simulink model "IeI"  (R2022a)
settings: Solver=FixedStepAuto  StartTime=0.0  StopTime=100000  FixedStep=0.01  RelTol=1e-3
libraries: cstblocks x3
settings Model: Creator=loryb  LastModifiedBy=loryb

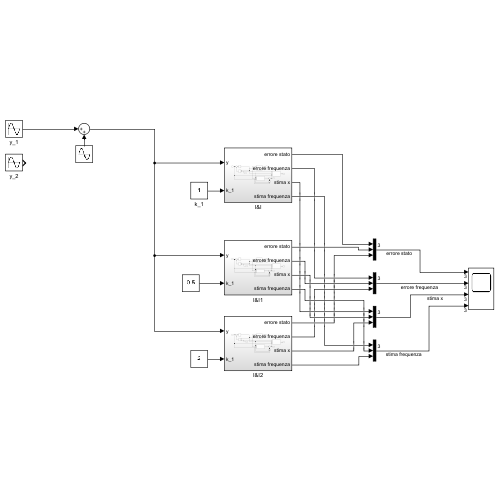
[thumbnail: Simulink's stored preview of the top-level diagram]
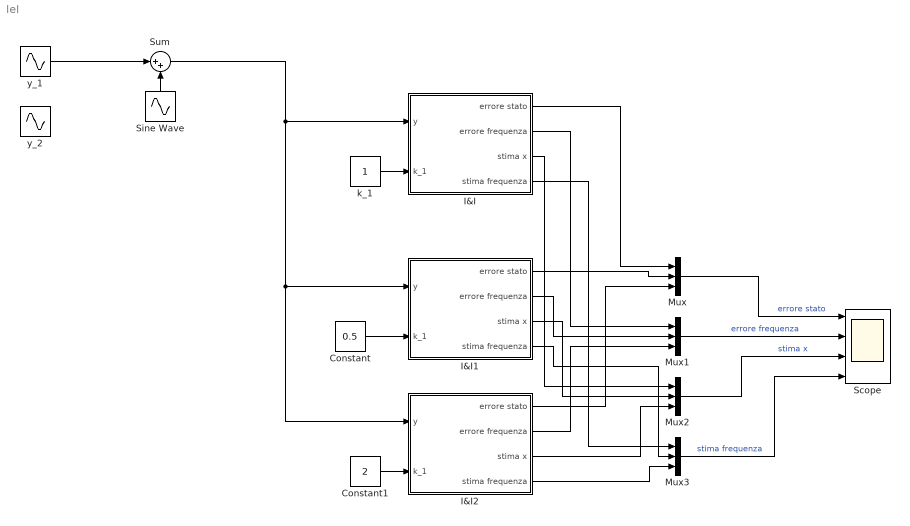
== system IeI ==
  Constant : Constant  Value=0.5
  Constant1 : Constant  Value=2
  I&I : Subsystem
  I&I1 : Subsystem
  I&I2 : Subsystem
  Mux{,1..3} (4 alike) : Mux  Inputs=3
  Scope : Scope  NumInputPorts=4
  Sine Wave : Sin  Amplitude=0.001  Frequency=50  SampleTime=0
  Sum : Sum  Inputs=|++
  k_1 : Constant
  y_1 : Sin  Frequency=100  SampleTime=0
  y_2 : Sin  SampleTime=0
  wires:
  Sum/1 -> I&I2/1(y), I&I1/1(y), I&I/1(y)
  k_1/1 -> I&I/2(k_1)
  Constant/1 -> I&I1/2(k_1)
  Constant1/1 -> I&I2/2(k_1)
  I&I/1(errore stato) -> Mux/1
  I&I1/1(errore stato) -> Mux/2
  I&I2/1(errore stato) -> Mux/3
  I&I/2(errore frequenza) -> Mux1/1
  I&I1/2(errore frequenza) -> Mux1/2
  I&I2/2(errore frequenza) -> Mux1/3
  I&I/3(stima x) -> Mux2/1
  I&I1/3(stima x) -> Mux2/2
  I&I2/3(stima x) -> Mux2/3
  I&I/4(stima frequenza) -> Mux3/1
  I&I1/4(stima frequenza) -> Mux3/2
  I&I2/4(stima frequenza) -> Mux3/3
  Mux/1 -> Scope/1  "errore stato"
  Mux1/1 -> Scope/2  "errore frequenza"
  Mux2/1 -> Scope/3  "stima x"
  Mux3/1 -> Scope/4  "stima frequenza"
  Sine Wave/1 -> Sum/2
  y_1/1 -> Sum/1

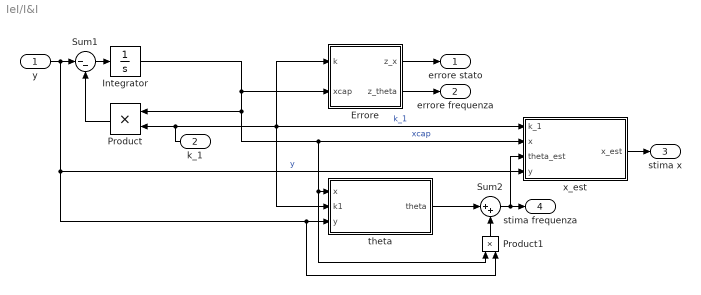
== system IeI/I&I ==
  y : Inport
  k_1 : Inport  Port=2
  Errore : Subsystem
  Integrator : Integrator
  Product : Product
  Product1 : Product
  Sum1 : Sum  Inputs=|--
  Sum2 : Sum  Inputs=|++
  theta : Subsystem
  x_est : Subsystem
  errore stato : Outport
  errore frequenza : Outport  Port=2
  stima x : Outport  Port=3
  stima frequenza : Outport  Port=4
  wires:
  Product/1 -> Sum1/2
  Sum1/1 -> Integrator/1
  k_1/1 -> theta/2(k1), Errore/1(k), x_est/1(k_1), Product/2  "k_1"
  Errore/1(z_x) -> errore stato/1
  Integrator/1 -> theta/1(x), Product1/1, x_est/2(x), Product/1, Errore/2(xcap)  "xcap"
  y/1 -> Product1/2, theta/3(y), x_est/4(y), Sum1/1  "y"
  Sum2/1 -> stima frequenza/1, x_est/3(theta_est)
  Product1/1 -> Sum2/2
  theta/1(theta) -> Sum2/1
  Errore/2(z_theta) -> errore frequenza/1
  x_est/1(x_est) -> stima x/1

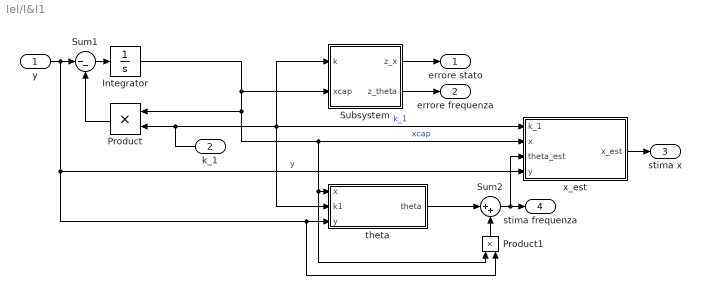
== system IeI/I&I1 ==
  y : Inport
  k_1 : Inport  Port=2
  Integrator : Integrator
  Product : Product
  Product1 : Product
  Subsystem : Subsystem
  Sum1 : Sum  Inputs=|--
  Sum2 : Sum  Inputs=|++
  theta : Subsystem
  x_est : Subsystem
  errore stato : Outport
  errore frequenza : Outport  Port=2
  stima x : Outport  Port=3
  stima frequenza : Outport  Port=4
  wires:
  Product/1 -> Sum1/2
  Sum1/1 -> Integrator/1
  k_1/1 -> theta/2(k1), Subsystem/1(k), x_est/1(k_1), Product/2  "k_1"
  Subsystem/1(z_x) -> errore stato/1
  Integrator/1 -> theta/1(x), Product1/1, x_est/2(x), Product/1, Subsystem/2(xcap)  "xcap"
  y/1 -> theta/3(y), Product1/2, x_est/4(y), Sum1/1  "y"
  Sum2/1 -> stima frequenza/1, x_est/3(theta_est)
  Product1/1 -> Sum2/2
  theta/1(theta) -> Sum2/1
  Subsystem/2(z_theta) -> errore frequenza/1
  x_est/1(x_est) -> stima x/1

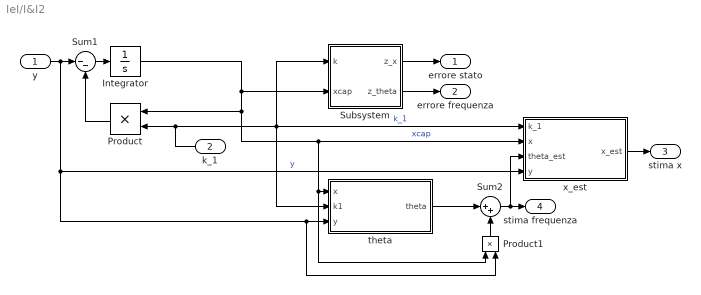
== system IeI/I&I2 ==
  y : Inport
  k_1 : Inport  Port=2
  Integrator : Integrator
  Product : Product
  Product1 : Product
  Subsystem : Subsystem
  Sum1 : Sum  Inputs=|--
  Sum2 : Sum  Inputs=|++
  theta : Subsystem
  x_est : Subsystem
  errore stato : Outport
  errore frequenza : Outport  Port=2
  stima x : Outport  Port=3
  stima frequenza : Outport  Port=4
  wires:
  Product/1 -> Sum1/2
  Sum1/1 -> Integrator/1
  k_1/1 -> theta/2(k1), Subsystem/1(k), x_est/1(k_1), Product/2  "k_1"
  Subsystem/1(z_x) -> errore stato/1
  Integrator/1 -> theta/1(x), Product1/1, x_est/2(x), Product/1, Subsystem/2(xcap)  "xcap"
  y/1 -> theta/3(y), Product1/2, x_est/4(y), Sum1/1  "y"
  Sum2/1 -> stima frequenza/1, x_est/3(theta_est)
  Product1/1 -> Sum2/2
  theta/1(theta) -> Sum2/1
  Subsystem/2(z_theta) -> errore frequenza/1
  x_est/1(x_est) -> stima x/1

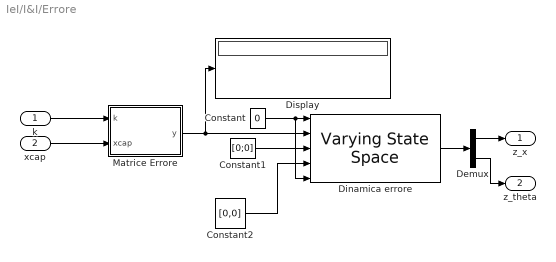
== system IeI/I&I/Errore ==
  k : Inport
  xcap : Inport  Port=2
  Constant : Constant  Value=0
  Constant1 : Constant  Value=[0;0]  VectorParams1D=off
  Constant2 : Constant  Value=[0,0]  VectorParams1D=off
  Demux : Demux  Outputs=2
  Dinamica errore : cstblocks/Linear Parameter Varying/Varying State Space  x0=1  xNames=''  OutputX=on  OutputDX=on
  Display : Display
  Matrice Errore : MATLAB Function  TreatAsAtomicUnit=on
  z_x : Outport
  z_theta : Outport  Port=2
  wires:
  k/1 -> Matrice Errore/1(k)
  xcap/1 -> Matrice Errore/2(xcap)
  Matrice Errore/1(y) -> Display/1, Dinamica errore/2
  Constant/1 -> Dinamica errore/5, Dinamica errore/1
  Constant1/1 -> Dinamica errore/3
  Constant2/1 -> Dinamica errore/4
  Dinamica errore/2 -> Demux/1
  Demux/1 -> z_x/1
  Demux/2 -> z_theta/1

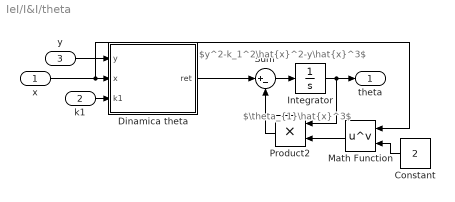
== system IeI/I&I/theta ==
  note: $\theta_{1}\hat{x}^3$
  note: $y^2-k_1^2\hat{x}^2-y\hat{x}^3$
  x : Inport
  k1 : Inport  Port=2
  y : Inport  Port=3
  Constant : Constant  Value=2
  Dinamica theta : MATLAB Function  TreatAsAtomicUnit=on
  Integrator : Integrator
  Math Function : Math  Operator=pow
  Product2 : Product
  Sum : Sum  Inputs=|+-
  theta : Outport
  wires:
  x/1 -> Math Function/1, Dinamica theta/2(x)
  Sum/1 -> Integrator/1
  Integrator/1 -> theta/1, Product2/1
  Product2/1 -> Sum/2
  Dinamica theta/1(ret) -> Sum/1
  y/1 -> Dinamica theta/1(y)
  k1/1 -> Dinamica theta/3(k1)
  Constant/1 -> Math Function/2
  Math Function/1 -> Product2/2

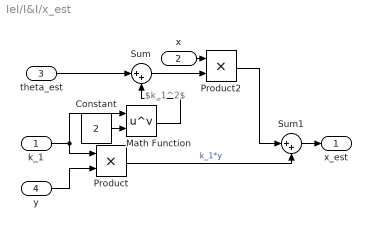
== system IeI/I&I/x_est ==
  note: $k_1^2$
  k_1 : Inport
  x : Inport  Port=2
  theta_est : Inport  Port=3
  y : Inport  Port=4
  Constant : Constant  Value=2
  Math Function : Math  Operator=pow
  Product : Product
  Product2 : Product
  Sum : Sum  Inputs=|++
  Sum1 : Sum  Inputs=|++
  x_est : Outport
  wires:
  y/1 -> Product/2
  k_1/1 -> Math Function/1, Product/1
  theta_est/1 -> Sum/1
  Math Function/1 -> Sum/2
  Sum/1 -> Product2/2
  x/1 -> Product2/1
  Sum1/1 -> x_est/1
  Product2/1 -> Sum1/1
  Product/1 -> Sum1/2  "k_1*y"
  Constant/1 -> Math Function/2

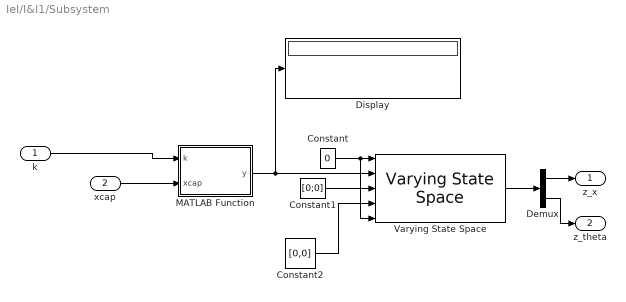
== system IeI/I&I1/Subsystem ==
  k : Inport
  xcap : Inport  Port=2
  Constant : Constant  Value=0
  Constant1 : Constant  Value=[0;0]  VectorParams1D=off
  Constant2 : Constant  Value=[0,0]  VectorParams1D=off
  Demux : Demux  Outputs=2
  Display : Display
  MATLAB Function : MATLAB Function  TreatAsAtomicUnit=on
  Varying State Space : cstblocks/Linear Parameter Varying/Varying State Space  x0=1  xNames=''  OutputX=on  OutputDX=on
  z_x : Outport
  z_theta : Outport  Port=2
  wires:
  k/1 -> MATLAB Function/1(k)
  xcap/1 -> MATLAB Function/2(xcap)
  MATLAB Function/1(y) -> Display/1, Varying State Space/2
  Constant/1 -> Varying State Space/5, Varying State Space/1
  Constant1/1 -> Varying State Space/3
  Constant2/1 -> Varying State Space/4
  Varying State Space/2 -> Demux/1
  Demux/1 -> z_x/1
  Demux/2 -> z_theta/1

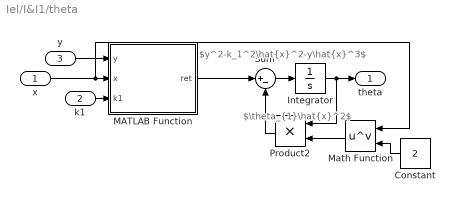
== system IeI/I&I1/theta ==
  note: $y^2-k_1^2\hat{x}^2-y\hat{x}^3$
  note: $\theta_{1}\hat{x}^2$
  x : Inport
  k1 : Inport  Port=2
  y : Inport  Port=3
  Constant : Constant  Value=2
  Integrator : Integrator
  MATLAB Function : MATLAB Function  TreatAsAtomicUnit=on
  Math Function : Math  Operator=pow
  Product2 : Product
  Sum : Sum  Inputs=|+-
  theta : Outport
  wires:
  Constant/1 -> Math Function/2
  Math Function/1 -> Product2/2
  Sum/1 -> Integrator/1
  Integrator/1 -> theta/1, Product2/1
  MATLAB Function/1(ret) -> Sum/1
  Product2/1 -> Sum/2
  k1/1 -> MATLAB Function/3(k1)
  x/1 -> Math Function/1, MATLAB Function/2(x)
  y/1 -> MATLAB Function/1(y)

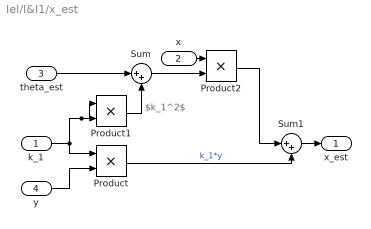
== system IeI/I&I1/x_est ==
  note: $k_1^2$
  k_1 : Inport
  x : Inport  Port=2
  theta_est : Inport  Port=3
  y : Inport  Port=4
  Product : Product
  Product1 : Product
  Product2 : Product
  Sum : Sum  Inputs=|++
  Sum1 : Sum  Inputs=|++
  x_est : Outport
  wires:
  y/1 -> Product/2
  k_1/1 -> Product1/1, Product1/2, Product/1
  theta_est/1 -> Sum/1
  Product1/1 -> Sum/2
  Sum/1 -> Product2/2
  x/1 -> Product2/1
  Sum1/1 -> x_est/1
  Product2/1 -> Sum1/1
  Product/1 -> Sum1/2  "k_1*y"

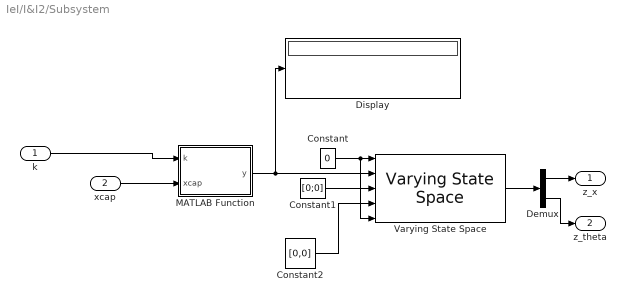
== system IeI/I&I2/Subsystem ==
  k : Inport
  xcap : Inport  Port=2
  Constant : Constant  Value=0
  Constant1 : Constant  Value=[0;0]  VectorParams1D=off
  Constant2 : Constant  Value=[0,0]  VectorParams1D=off
  Demux : Demux  Outputs=2
  Display : Display
  MATLAB Function : MATLAB Function  TreatAsAtomicUnit=on
  Varying State Space : cstblocks/Linear Parameter Varying/Varying State Space  x0=1  xNames=''  OutputX=on  OutputDX=on
  z_x : Outport
  z_theta : Outport  Port=2
  wires:
  k/1 -> MATLAB Function/1(k)
  xcap/1 -> MATLAB Function/2(xcap)
  MATLAB Function/1(y) -> Display/1, Varying State Space/2
  Constant/1 -> Varying State Space/5, Varying State Space/1
  Constant1/1 -> Varying State Space/3
  Constant2/1 -> Varying State Space/4
  Varying State Space/2 -> Demux/1
  Demux/1 -> z_x/1
  Demux/2 -> z_theta/1

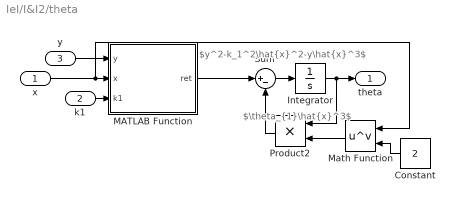
== system IeI/I&I2/theta ==
  note: $y^2-k_1^2\hat{x}^2-y\hat{x}^3$
  note: $\theta_{1}\hat{x}^3$
  x : Inport
  k1 : Inport  Port=2
  y : Inport  Port=3
  Constant : Constant  Value=2
  Integrator : Integrator
  MATLAB Function : MATLAB Function  TreatAsAtomicUnit=on
  Math Function : Math  Operator=pow
  Product2 : Product
  Sum : Sum  Inputs=|+-
  theta : Outport
  wires:
  Constant/1 -> Math Function/2
  Math Function/1 -> Product2/2
  Sum/1 -> Integrator/1
  Integrator/1 -> theta/1, Product2/1
  MATLAB Function/1(ret) -> Sum/1
  Product2/1 -> Sum/2
  k1/1 -> MATLAB Function/3(k1)
  x/1 -> Math Function/1, MATLAB Function/2(x)
  y/1 -> MATLAB Function/1(y)

== system IeI/I&I2/x_est ==
  note: $k_1^2$
  k_1 : Inport
  x : Inport  Port=2
  theta_est : Inport  Port=3
  y : Inport  Port=4
  Product : Product
  Product1 : Product
  Product2 : Product
  Sum : Sum  Inputs=|++
  Sum1 : Sum  Inputs=|++
  x_est : Outport
  wires:
  y/1 -> Product/2
  k_1/1 -> Product1/1, Product1/2, Product/1
  theta_est/1 -> Sum/1
  Product1/1 -> Sum/2
  Sum/1 -> Product2/2
  x/1 -> Product2/1
  Sum1/1 -> x_est/1
  Product2/1 -> Sum1/1
  Product/1 -> Sum1/2  "k_1*y"

== matlab function IeI/I&I/Errore/Matrice Errore ==
  data: k input; y output; xcap input
function y = fcn(k,xcap)
m=-ones(2,2);
m(1,1)=m(1,1)*abs(k);
m(1,2)=0;
m(2,1)=m(2,1)*xcap;
m(2,2)=m(2,2)*xcap*xcap;
y = m;

== matlab function IeI/I&I1/Subsystem/MATLAB Function ==
  data: k input; y output; xcap input
function y = fcn(k,xcap)
m=-ones(2,2);
m(1,1)=m(1,1)*abs(k);
m(1,2)=0;
m(2,1)=m(2,1)*xcap;
m(2,2)=m(2,2)*xcap*xcap;
y = m;

== matlab function IeI/I&I1/theta/MATLAB Function ==
  data: y input; ret output; x input; k1 input
function ret = fcn(y,x,k1)

ret = y^2-k1^2*x^2-y*x^3;

== matlab function IeI/I&I2/Subsystem/MATLAB Function ==
  data: k input; y output; xcap input
function y = fcn(k,xcap)
m=-ones(2,2);
m(1,1)=m(1,1)*abs(k);
m(1,2)=0;
m(2,1)=m(2,1)*xcap;
m(2,2)=m(2,2)*xcap*xcap;
y = m;

== matlab function IeI/I&I2/theta/MATLAB Function ==
  data: y input; ret output; x input; k1 input
function ret = fcn(y,x,k1)

ret = y^2-k1^2*x^2-y*x^3;

== matlab function IeI/I&I/theta/Dinamica theta ==
  data: y input; ret output; x input; k1 input
function ret = fcn(y,x,k1)

ret = y^2-k1^2*x^2-y*x^3;
